simulink model "unicycle_regulation_pose"  (R2025b)
settings: Solver=ode5  StartTime=0.0  StopTime=15  FixedStep=1e-3  RelTol=1e-3
settings Model: Creator=Cris  LastModifiedBy=Cris

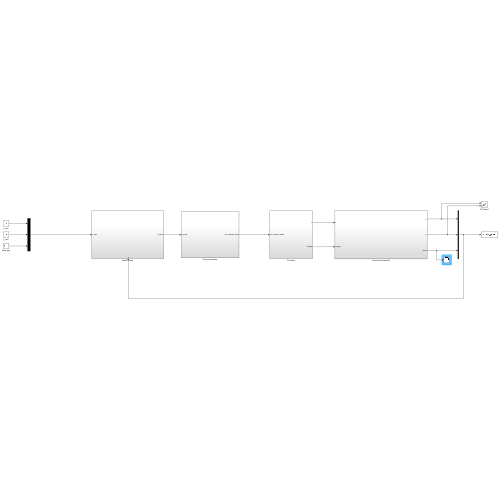
[thumbnail: Simulink's stored preview of the top-level diagram]
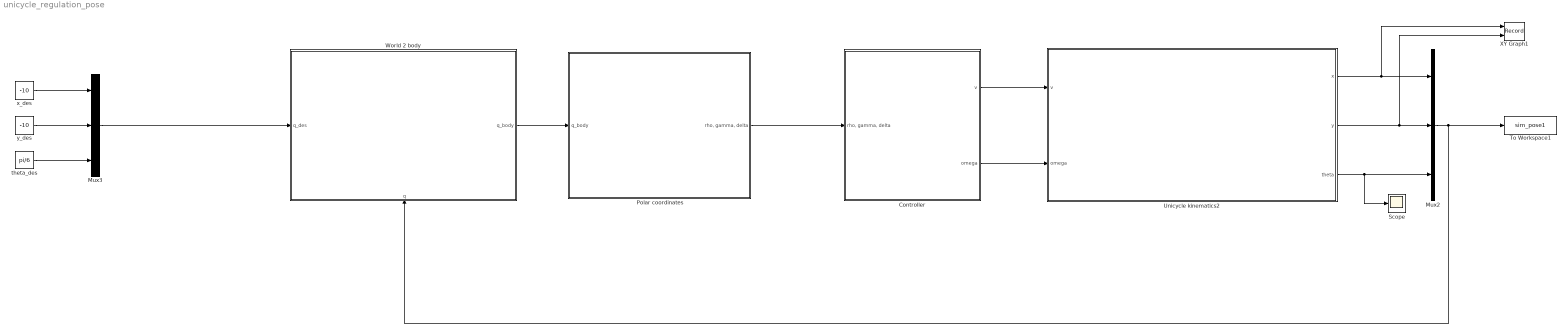
== system unicycle_regulation_pose ==
  Controller : Subsystem
  Mux2 : Mux  Inputs=3
  Mux3 : Mux  Inputs=3
  Polar coordinates : Subsystem
  Scope : Scope
      settings: ActiveDisplayYMinimum=-3.6435767001594175  ActiveDisplayYMaximum=1.2956769953230405
  To Workspace1 : ToWorkspace  VariableName=sim_pose1  SaveFormat=Timeseries  SampleTime=-1
  Unicycle kinematics2 : Subsystem
  World 2 body : Subsystem
      settings: PortSchema="{\"entries\":[{\"content\":{\"sides\":[{\"content\":{\"connectorIds\":[\"In1\"]},\"type\":\"ConnectorPlacement.EquallySpacedRectSide\",\"uuid\":\"d6332ee4-6e37-4568-865c-a04eee2f5a67\"},{\"content\":{\"connectorIds\":[\"Out1\"],\"side\":\"RIGHT\"},\"type\":\"ConnectorPlacement.EquallySpacedRectSide\",\"uuid\":\"8e88a442-f659-4873-b48a-1ad3acef8f2e\"},{\"content\":{\"side\":\"TOP\"},\"type\":\"ConnectorPlacement.EquallySpacedRectSide\",\"uuid\":\"5470688b-b468-4d37-81dc-c9eceb17c0d6\"},{\"content\":{\"connectorIds\":[\"In2\"],\"side\":\"BOTTOM\"},\"type\":\"ConnectorPlacement.EquallySpacedRectSide\",\"uuid\":\"59461b8c-7911-43ca-b37e-6874a62a6425\"}]},\"type\":\"ConnectorPlacement.EquallySpacedConnector\",\"uuid\":\"674f477f-0e86-4671-9466-4d2b04f4aa78\"}],\"packageUris\":[\"http://schema.mathworks.com/mf0/Connector/R2020b\"],\"version\":\"1.0\"}"
  XY Graph1 : Record  NumPorts=2.0  FileSettingsInternal="{\"entries\":[{\"content\":{\"excelSettings\":{\"content\":{},\"type\":\"Streamout.ExcelSettings\"},\"parquetSettings\":{\"content\":{},\"type\":\"Streamout.ParquetSettings\"}},\"type\":\"Streamout.FileSettingStorage\",\"uuid\":\"\"}],\"packageUris\":[\"http:\\/\\/schema.mathworks.com\\/mf0\\/streamout_blocks\\/R2020a\"],\"version\":\"1.0\"}"  FrameSettings=[0, 0]  Layout=[1 1]  SignalsInternal="{\"entries\":[{\"content\":{\"signals\":[{\"content\":{\"blockPath\":[],\"dimensions\":[1],\"domain\":\"\",\"lineColor\":\"#a2142f\",\"plots\":[ 1 ],\"port\":1,\"sid\":[\"\"],\"signalID\":1,\"signalName\":\"Unicycle kinematics2:1\"},\"type\":\"RecordBlkView.Signal\",\"uuid\":\"\"},{\"content\":{\"blockPath\":[],\"dimensions\":[1],\"domain\":\"\",\"lineColor\":\"#139fff\",\"plots\":[ 1 ],\"port\":2,\"sid\":[\"\"],\"signalID\":2,\"signalName\":\"Unicycle kinematics2:2\"},\"type\":\"RecordBlkView.Signal\",\"uuid\":\"\"}]},\"type\":\"RecordBlkView.InputSignals\",\"uuid\":\"\"}],\"packageUris\":[\"http:\\/\\/schema.mathworks.com\\/mf0\\/streamout_blocks\\/R2020a\"],\"version\":\"1.0\"}"  VisualizationBindings="{\"xyplotplugin\":{\"info\":[{\"series\":[{\"bindingParametersList\":[{\"parameter\":\"X-Axis\",\"signalID\":1,\"signalName\":\"Unicycle kinematics2:1\"},{\"parameter\":\"Y-Axis\",\"signalID\":2,\"signalName\":\"Unicycle kinematics2:2\"}],\"seriesID\":0}],\"subplotID\":1}]}}"  CompatibilityTag=XY
  theta_des : Constant  Value=pi/6
  x_des : Constant  Value=-10
  y_des : Constant  Value=-10
  wires:
  y_des/1 -> Mux3/2
  x_des/1 -> Mux3/1
  theta_des/1 -> Mux3/3
  Mux3/1 -> World 2 body/1(q_des)
  World 2 body/1(q_body) -> Polar coordinates/1(q_body)
  Polar coordinates/1("rho, gamma, delta") -> Controller/1("rho, gamma, delta")
  Controller/1(v) -> Unicycle kinematics2/1(v)
  Controller/2(omega) -> Unicycle kinematics2/2(omega)
  Unicycle kinematics2/1(x) -> XY Graph1/1, Mux2/1
  Unicycle kinematics2/2(y) -> Mux2/2, XY Graph1/2
  Unicycle kinematics2/3(theta) -> Mux2/3, Scope/1
  Mux2/1 -> To Workspace1/1, World 2 body/2(q)

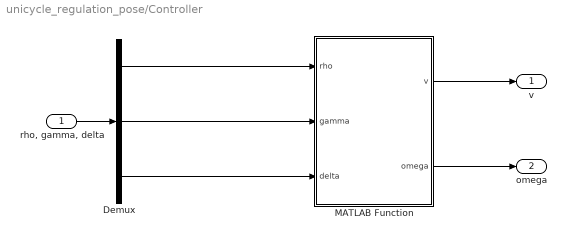
== system unicycle_regulation_pose/Controller ==
  "rho, gamma, delta" : Inport
  Demux : Demux  Outputs=3
  MATLAB Function : MATLAB Function  TreatAsAtomicUnit=on
  v : Outport
  omega : Outport  Port=2
  wires:
  "rho, gamma, delta"/1 -> Demux/1
  Demux/1 -> MATLAB Function/1(rho)
  Demux/2 -> MATLAB Function/2(gamma)
  Demux/3 -> MATLAB Function/3(delta)
  MATLAB Function/1(v) -> v/1
  MATLAB Function/2(omega) -> omega/1

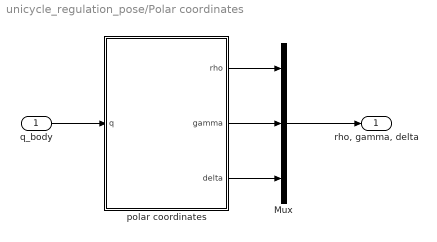
== system unicycle_regulation_pose/Polar coordinates ==
  q_body : Inport
  Mux : Mux  Inputs=3
  polar coordinates : MATLAB Function  TreatAsAtomicUnit=on
  "rho, gamma, delta" : Outport
  wires:
  q_body/1 -> polar coordinates/1(q)
  polar coordinates/1(rho) -> Mux/1
  polar coordinates/2(gamma) -> Mux/2
  polar coordinates/3(delta) -> Mux/3
  Mux/1 -> "rho, gamma, delta"/1

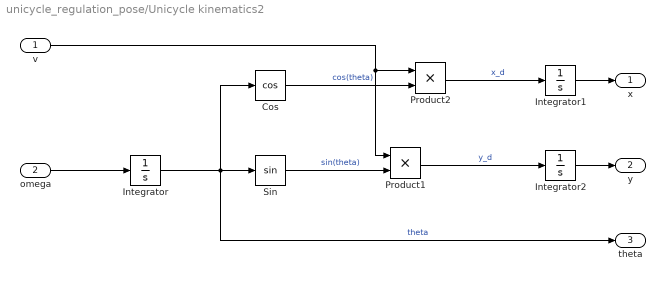
== system unicycle_regulation_pose/Unicycle kinematics2 ==
  v : Inport
  omega : Inport  Port=2
  Cos : Trigonometry  Operator=cos
  Integrator : Integrator
  Integrator1 : Integrator
  Integrator2 : Integrator
  Product1 : Product
  Product2 : Product
  Sin : Trigonometry
  x : Outport
  y : Outport  Port=2
  theta : Outport  Port=3
  wires:
  omega/1 -> Integrator/1
  Integrator/1 -> theta/1, Cos/1, Sin/1  "theta"
  Cos/1 -> Product2/2  "cos(theta)"
  Sin/1 -> Product1/2  "sin(theta)"
  v/1 -> Product2/1, Product1/1
  Integrator1/1 -> x/1
  Product2/1 -> Integrator1/1  "x_d"
  Integrator2/1 -> y/1
  Product1/1 -> Integrator2/1  "y_d"

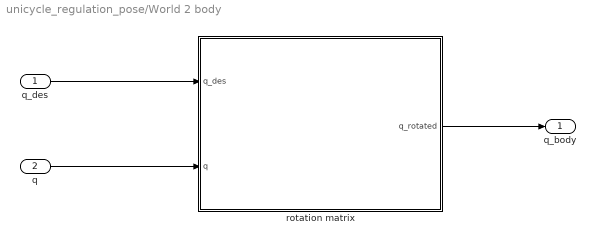
== system unicycle_regulation_pose/World 2 body ==
  q_des : Inport
  q : Inport  Port=2
  rotation matrix : MATLAB Function  TreatAsAtomicUnit=on
  q_body : Outport
  wires:
  q/1 -> rotation matrix/2(q)
  q_des/1 -> rotation matrix/1(q_des)
  rotation matrix/1(q_rotated) -> q_body/1

== matlab function unicycle_regulation_pose/World 2 body/rotation matrix ==
  data: q_des input; q input; q_rotated output
function q_rotated  = fcn(q_des, q)

theta_des = q_des(3);

% rotation matrix
R = [cos(theta_des), sin(theta_des), 0;
    -sin(theta_des), cos(theta_des), 0; 
    0,              0,              1];

% rotate
delta_q = q - q_des;
q_rotated = R*delta_q;

== matlab function unicycle_regulation_pose/Polar coordinates/polar coordinates ==
  data: q input; rho output; gamma output; delta output
function [rho, gamma, delta] = fcn(q)

%auxiliary
dx = q(1);
dy = q(2);
dtheta = q(3);

% trasformation in polar coordinates
rho = sqrt(dx^2+dy^2);
gamma = atan2(-dy, -dx) - dtheta;
delta = atan2(-dy, -dx);

% !!!!!!!!!!!!!!!!!!!!!!!!Normalize angles to [-pi, pi]
gamma = atan2(sin(gamma), cos(gamma));
delta = atan2(sin(delta), cos(delta));

== matlab function unicycle_regulation_pose/Controller/MATLAB Function ==
  data: v output; rho input; gamma input; omega output; delta input
function [v , omega] = fcn(rho, gamma, delta)

% adjust gains
k1 = 2;
k2 = 3;
k3 = 5;


% controller

v = k1*rho*cos(gamma);

if (abs(sin(gamma)/gamma) > 0.001)
    temp = sin(gamma)/gamma;
else
    temp = 1;
end

omega = k2*gamma + (k1*temp*cos(gamma))*(gamma+k3*delta);
